simulink model "closed_loop_sim"  (R2022b)
settings: Solver=ode4  StartTime=0.0  StopTime=10.0  FixedStep=0.001  RelTol=1e-3
values from neighbouring files (symbols this model uses):
  state_init = [ vx_init; vy_init; r_init; x_pos_init; y_pos_init; angle_init]    [drift_sim.m]
settings Model: Creator=malac  LastModifiedBy=malac

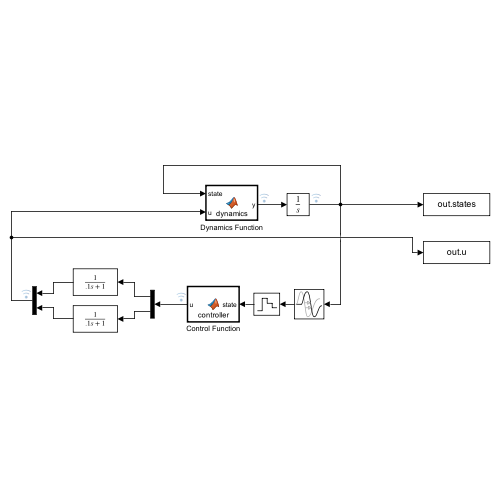
[thumbnail: Simulink's stored preview of the top-level diagram]
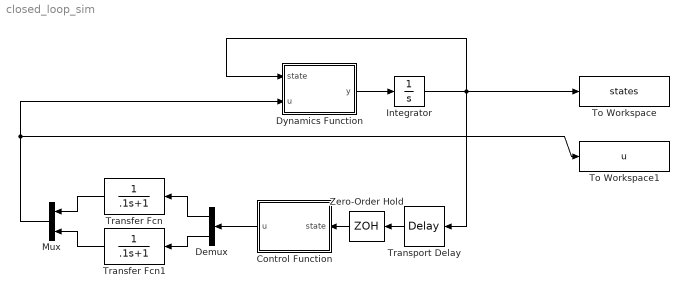
== system closed_loop_sim ==
  Control Function : MATLAB Function  TreatAsAtomicUnit=on
  Demux : Demux  Outputs=2
  Dynamics Function : MATLAB Function  TreatAsAtomicUnit=on
  Integrator : Integrator  InitialCondition=[state_init]
  Mux : Mux  Inputs=2
  To Workspace : ToWorkspace  VariableName=states  SaveFormat=Timeseries  SampleTime=-1
  To Workspace1 : ToWorkspace  VariableName=u  SaveFormat=Timeseries  SampleTime=-1
  Transfer Fcn : TransferFcn  Denominator=[.1 1]
  Transfer Fcn1 : TransferFcn  Denominator=[.1 1]
  Transport Delay : TransportDelay  DelayTime=.005
  Zero-Order Hold : ZeroOrderHold  SampleTime=0.05
  wires:
  Dynamics Function/1(y) -> Integrator/1
  Zero-Order Hold/1 -> Control Function/1(state)
  Integrator/1 -> Dynamics Function/1(state), To Workspace/1, Transport Delay/1
  Transport Delay/1 -> Zero-Order Hold/1
  Mux/1 -> To Workspace1/1, Dynamics Function/2(u)
  Transfer Fcn1/1 -> Mux/2
  Transfer Fcn/1 -> Mux/1
  Demux/1 -> Transfer Fcn/1
  Demux/2 -> Transfer Fcn1/1
  Control Function/1(u) -> Demux/1

== matlab function closed_loop_sim/Dynamics Function ==
  data: y output; state input; u input
function y = dynamics(state, u)
    % Parameters of RC car in paper, probably a good place to start
    m = 2.04;       % Mass [kg]
    Lr = .1087;     % Distance from CM to rear axle [m]
    Lf = .1513;     % Distance from CM to front axle [m]
    Iz = 0.03;      % Yaw moment of inertia [kg/m^2]
    Cr = 127.77;    % Rear tire cornering stiffness
    Cf = 47.86;     % Front tire cornering stiffness
    mu_r = 0.33;    % Rear tire coefficient of friction
    mu_f = 0.35;    % Front tire coefficient of friction
    g = 9.81;       % Acceleration due to gravity [m/s^2]

    vx = state(1);
    vy = state(2);
    r = state(3);
    x_pos = state(4);
    y_pos = state(5);
    yaw_angle = state(6);
   
    vx_inertial = vx*cos(yaw_angle)- vy*sin(yaw_angle);
    vy_inertial = vx*sin(yaw_angle)+ vy*cos(yaw_angle);

    y = [drift_eom(0, [vx, vy, r], u, g, Lf, Lr, m, Iz, Cr, Cf, mu_r, mu_f); vx_inertial; vy_inertial; r];

== matlab function closed_loop_sim/Control Function ==
  data: u output; state input
function u = controller(state)

    u = drift_LQR_controller(state(1:3));
